simulink model "lab11"  (R2014b)
settings: Solver=ode45  StartTime=0.0  StopTime=25.0  MaxStep=0.001  MinStep=0.0001  RelTol=1e-3
values from neighbouring files (symbols this model uses):
  Cp = 0.5*10^8    (= 50000000)    [Lab11.m]
  Kd = 0.9*10^3    (= 900)    [Lab11.m]
  Ko = 8.2    [Lab11.m]
  m = 0.3    [Lab11.m]
  Tu = 0.06    [Lab11.m]
undefined symbols (not defined in the file or in its folder): Kf, Ku, Kv, Kx
settings Model: Creator=Игорь  LastModifiedBy=Игорь

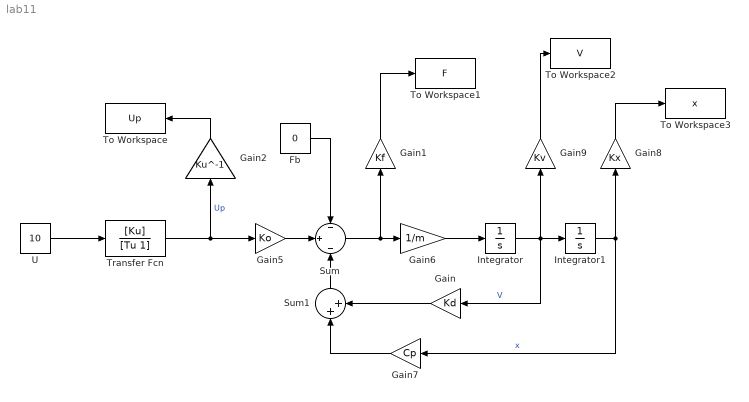
== system lab11 ==
  Fb : Constant  Value=0
  Gain : Gain  Gain=Kd
  Gain1 : Gain  Gain=Kf
  Gain2 : Gain  Gain=Ku^-1
  Gain5 : Gain  Gain=Ko
  Gain6 : Gain  Gain=1/m
  Gain7 : Gain  Gain=Cp
  Gain8 : Gain  Gain=Kx
  Gain9 : Gain  Gain=Kv
  Integrator : Integrator
  Integrator1 : Integrator
  Sum : Sum  Inputs=-|+|-
  Sum1 : Sum  Inputs=|++
  To Workspace : ToWorkspace  VariableName=Up  SaveFormat=Timeseries  SampleTime=-1
  To Workspace1 : ToWorkspace  VariableName=F  SaveFormat=Timeseries  SampleTime=-1
  To Workspace2 : ToWorkspace  VariableName=V  SaveFormat=Timeseries  SampleTime=-1
  To Workspace3 : ToWorkspace  VariableName=x  SaveFormat=Timeseries  SampleTime=-1
  Transfer Fcn : TransferFcn  Numerator=[Ku]  Denominator=[Tu 1]
  U : Constant  Value=10
  wires:
  Transfer Fcn/1 -> Gain5/1, Gain2/1  "Up"
  Gain5/1 -> Sum/2
  Integrator/1 -> Gain/1, Integrator1/1, Gain9/1  "V"
  Gain6/1 -> Integrator/1
  Sum/1 -> Gain6/1, Gain1/1
  Gain/1 -> Sum1/2
  Sum1/1 -> Sum/3
  Integrator1/1 -> Gain7/1, Gain8/1  "x"
  Gain7/1 -> Sum1/1
  U/1 -> Transfer Fcn/1
  Fb/1 -> Sum/1
  Gain2/1 -> To Workspace/1
  Gain8/1 -> To Workspace3/1
  Gain9/1 -> To Workspace2/1
  Gain1/1 -> To Workspace1/1
